simulink subsystem "s_tx_uart"  (R2024b)
settings: Solver=VariableStepAuto  StartTime=0.0  StopTime=10.0  RelTol=1e-3
undefined symbols (not defined in the file): A0, A1, PTB2, PTB3
libraries: frdmk64flib x3, etargetslib x2
settings Model: Creator=marwa  LastModifiedBy=marwa

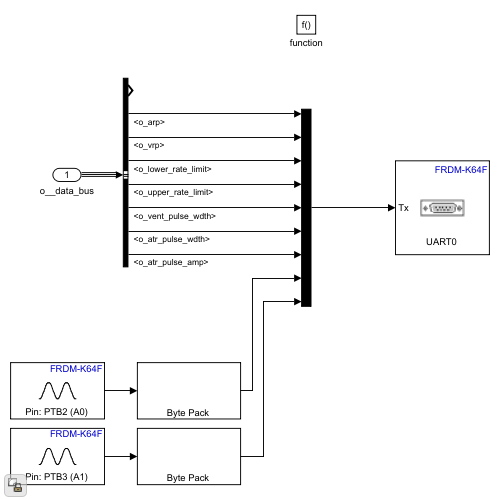
[thumbnail: Simulink's stored preview of the top-level diagram]
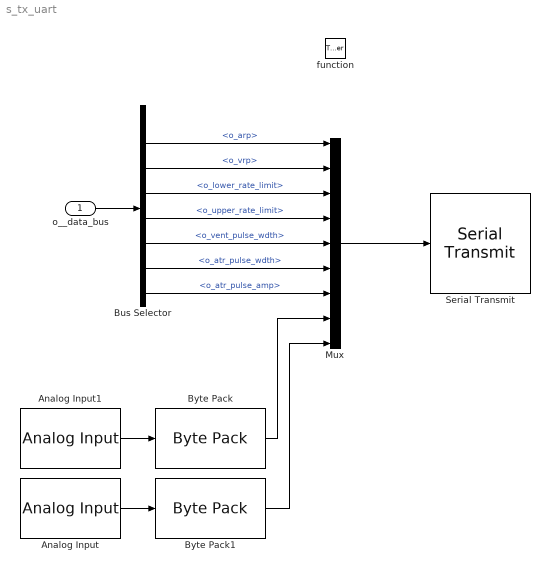
== system s_tx_uart ==
  o__data_bus : Inport
  function : TriggerPort  TriggerType=function-call  FunctionName=drive_outputs  VariantControl=(inherit)
  Analog Input : frdmk64flib/Analog Input  Whichpin=PTB3 (A1)  SampleTime=-1
  Analog Input1 : frdmk64flib/Analog Input  Whichpin=PTB2 (A0)  SampleTime=-1
  Bus Selector : BusSelector  OutputSignals=o_mode,o_arp,o_vrp,o_lower_rate_limit,o_upper_rate_limit,o_vent_pulse_wdth,o_atr_pulse_wdth,o_atr_pulse_amp
  Byte Pack : etargetslib/Byte Pack  datatypes={'double'}  byteAlign=1
  Byte Pack1 : etargetslib/Byte Pack  datatypes={'double'}  byteAlign=1
  Mux : Mux  Inputs=9
  Serial Transmit : frdmk64flib/Serial Transmit  SCIModule=0  Baudrate=uint32(9600)  Parity=None  StopBits=1  HardwareFlowControl=None  ByteOrder=LittleEndian  BlockingMode=on  OutputStatus=off
  wires:
  Byte Pack/1 -> Mux/8
  Analog Input1/1 -> Byte Pack/1
  Bus Selector/6 -> Mux/5  "<o_vent_pulse_wdth>"
  Bus Selector/8 -> Mux/7  "<o_atr_pulse_amp>"
  Bus Selector/7 -> Mux/6  "<o_atr_pulse_wdth>"
  Bus Selector/4 -> Mux/3  "<o_lower_rate_limit>"
  o__data_bus/1 -> Bus Selector/1
  Mux/1 -> Serial Transmit/1
  Bus Selector/3 -> Mux/2  "<o_vrp>"
  Bus Selector/5 -> Mux/4  "<o_upper_rate_limit>"
  Analog Input/1 -> Byte Pack1/1
  Bus Selector/2 -> Mux/1  "<o_arp>"
  Byte Pack1/1 -> Mux/9
